simulink model "MdLCtrl_IPC"  (R2019a)
settings: Solver=FixedStepAuto  StartTime=0.0  StopTime=10.0  RelTol=1e-3
values from neighbouring files (symbols this model uses):
  Control = 0.0    [DD_CtrlBaseline.sldd]    (also in DD_MdlCtrl_qLPVMPC.sldd = 0.0
  P_InitAngle = 0.106    [DD_CtrlBaseline.sldd]    (also in ctrl_data.m)
undefined symbols (not defined in the file or in its folder): c1, c2, d1, d2, d3, IPC_An, IPC_K_1P, IPC_KI_1p, IPC_KP_1p, kp_Turm, offest_1p, T_Turmfilter, v_Gen_nenn
settings Model: Creator=ditt_aj  LastModifiedBy=ditt_aj

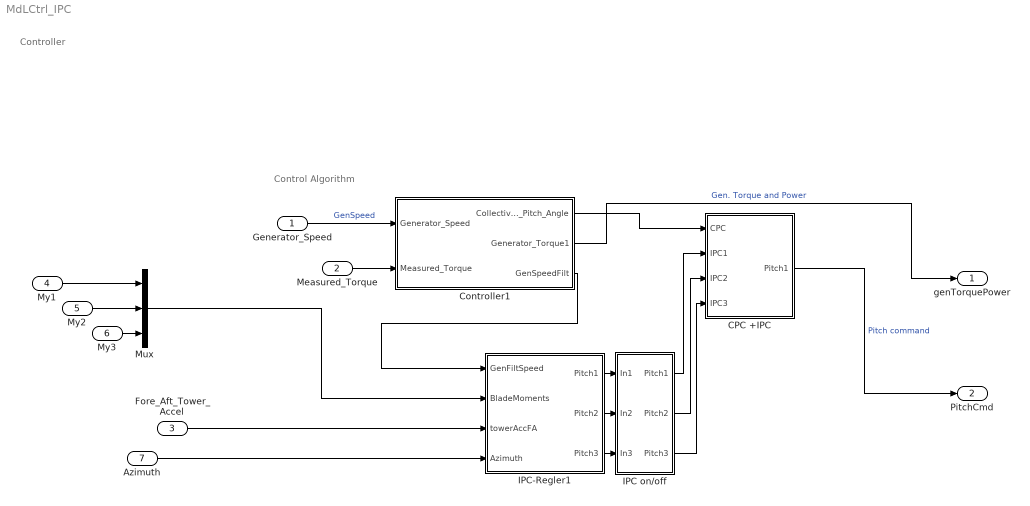
== system MdLCtrl_IPC ==
  note: Control Algorithm
  note: Controller
  Generator_Speed : Inport
  Measured_Torque : Inport  Port=2
  Fore_Aft_Tower_Accel : Inport  Port=3
  My1 : Inport  Port=4
  My2 : Inport  Port=5
  My3 : Inport  Port=6
  Azimuth : Inport  Port=7
  CPC +IPC : Subsystem
  Controller1 : Subsystem
  IPC on/off : Subsystem
  IPC-Regler1 : Subsystem
  Mux : Mux  Inputs=3
  genTorquePower : Outport
  PitchCmd : Outport  Port=2
  wires:
  CPC +IPC/1(Pitch1) -> PitchCmd/1  "Pitch command"
  Controller1/2(Generator_Torque1) -> genTorquePower/1  "Gen. Torque and Power"
  My1/1 -> Mux/1
  My2/1 -> Mux/2
  My3/1 -> Mux/3
  Generator_Speed/1 -> Controller1/1(Generator_Speed)  "GenSpeed"
  Fore_Aft_Tower_Accel/1 -> IPC-Regler1/3(towerAccFA)
  Mux/1 -> IPC-Regler1/2(BladeMoments)
  Azimuth/1 -> IPC-Regler1/4(Azimuth)
  IPC-Regler1/2(Pitch2) -> IPC on/off/2(In2)
  IPC-Regler1/1(Pitch1) -> IPC on/off/1(In1)
  IPC-Regler1/3(Pitch3) -> IPC on/off/3(In3)
  IPC on/off/2(Pitch2) -> CPC +IPC/3(IPC2)
  Controller1/1(Collective_Pitch_Angle) -> CPC +IPC/1(CPC)
  IPC on/off/1(Pitch1) -> CPC +IPC/2(IPC1)
  Controller1/3(GenSpeedFilt) -> IPC-Regler1/1(GenFiltSpeed)
  IPC on/off/3(Pitch3) -> CPC +IPC/4(IPC3)
  Measured_Torque/1 -> Controller1/2(Measured_Torque)

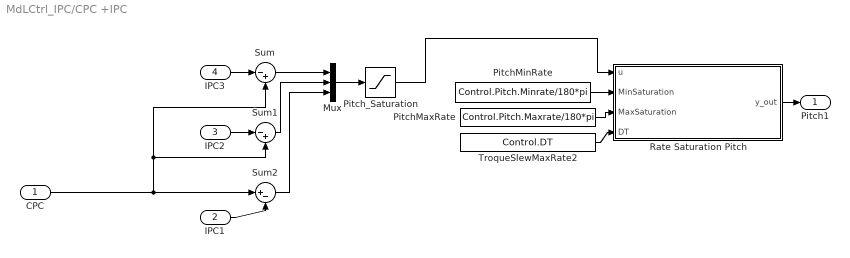
== system MdLCtrl_IPC/CPC +IPC ==
  CPC : Inport
  IPC1 : Inport  Port=2
  IPC2 : Inport  Port=3
  IPC3 : Inport  Port=4
  Mux : Mux  Inputs=3
  PitchMaxRate : Constant  Value=Control.Pitch.Maxrate/180*pi
  PitchMinRate : Constant  Value=Control.Pitch.Minrate/180*pi
  Pitch_Saturation : Saturate  UpperLimit=Control.Pitch.Max*pi/180  LowerLimit=Control.Pitch.Min*pi/180
  Rate Saturation Pitch : MATLAB Function  TreatAsAtomicUnit=on
  Sum : Sum  Inputs=|-+
  Sum1 : Sum  Inputs=|-+
  Sum2 : Sum  Inputs=|+-
  TroqueSlewMaxRate2 : Constant  Value=Control.DT
  Pitch1 : Outport
  wires:
  IPC3/1 -> Sum/1
  IPC2/1 -> Sum1/1
  IPC1/1 -> Sum2/2
  CPC/1 -> Sum1/2, Sum/2, Sum2/1
  TroqueSlewMaxRate2/1 -> Rate Saturation Pitch/4(DT)
  Mux/1 -> Pitch_Saturation/1
  Pitch_Saturation/1 -> Rate Saturation Pitch/1(u)
  PitchMaxRate/1 -> Rate Saturation Pitch/3(MaxSaturation)
  PitchMinRate/1 -> Rate Saturation Pitch/2(MinSaturation)
  Sum/1 -> Mux/1
  Sum1/1 -> Mux/2
  Sum2/1 -> Mux/3
  Rate Saturation Pitch/1(y_out) -> Pitch1/1

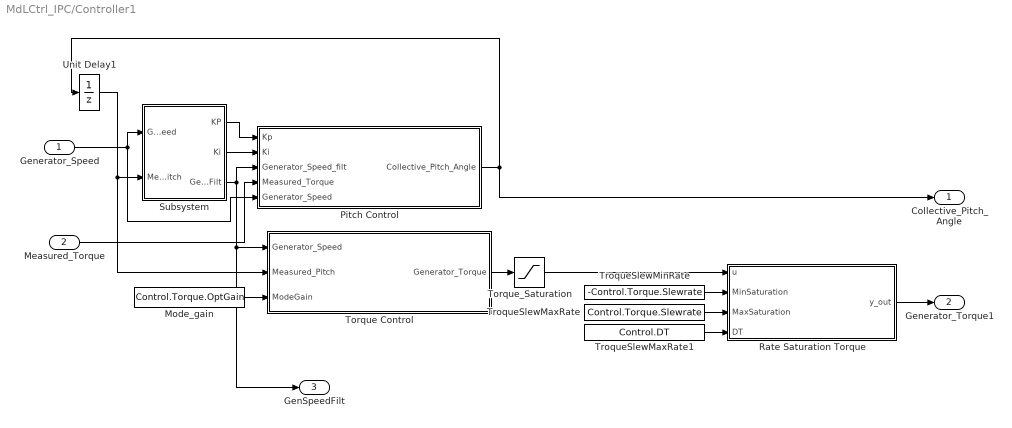
== system MdLCtrl_IPC/Controller1 ==
  Generator_Speed : Inport
  Measured_Torque : Inport  Port=2
  Mode_gain : Constant  Value=Control.Torque.OptGain
  Pitch Control : Subsystem
  Rate Saturation Torque : MATLAB Function  TreatAsAtomicUnit=on
  Subsystem : Subsystem
  Torque Control : Subsystem
  Torque_Saturation : Saturate  UpperLimit=Control.Torque.Limit  LowerLimit=Control.Torque.Min
  TroqueSlewMaxRate : Constant  Value=Control.Torque.Slewrate
  TroqueSlewMaxRate1 : Constant  Value=Control.DT
  TroqueSlewMinRate : Constant  Value=-Control.Torque.Slewrate
  Unit Delay1 : UnitDelay  InitialCondition=P_InitAngle*pi/180  SampleTime=-1  HasFrameUpgradeWarning=on
  Collective_Pitch_Angle : Outport
  Generator_Torque1 : Outport  Port=2
  GenSpeedFilt : Outport  Port=3
  wires:
  Mode_gain/1 -> Torque Control/3(ModeGain)
  Torque_Saturation/1 -> Rate Saturation Torque/1(u)
  TroqueSlewMinRate/1 -> Rate Saturation Torque/2(MinSaturation)
  TroqueSlewMaxRate/1 -> Rate Saturation Torque/3(MaxSaturation)
  TroqueSlewMaxRate1/1 -> Rate Saturation Torque/4(DT)
  Torque Control/1(Generator_Torque) -> Torque_Saturation/1
  Rate Saturation Torque/1(y_out) -> Generator_Torque1/1
  Pitch Control/1(Collective_Pitch_Angle) -> Unit Delay1/1, Collective_Pitch_Angle/1
  Generator_Speed/1 -> Pitch Control/5(Generator_Speed), Subsystem/1(GenSpeed)
  Unit Delay1/1 -> Torque Control/2(Measured_Pitch), Subsystem/2(MesasuredPitch)
  Subsystem/3(GenSpeedFilt) -> GenSpeedFilt/1, Torque Control/1(Generator_Speed), Pitch Control/3(Generator_Speed_filt)
  Subsystem/1(KP) -> Pitch Control/1(Kp)
  Subsystem/2(Ki) -> Pitch Control/2(Ki)
  Measured_Torque/1 -> Pitch Control/4(Measured_Torque)

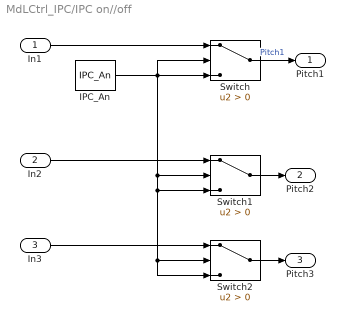
== system MdLCtrl_IPC/IPC on//off ==
  In1 : Inport
  In2 : Inport  Port=2
  In3 : Inport  Port=3
  IPC_An : Constant  Value=IPC_An
  Switch : Switch  Criteria=u2 > Threshold
  Switch1 : Switch  Criteria=u2 > Threshold
  Switch2 : Switch  Criteria=u2 > Threshold
  Pitch1 : Outport
  Pitch2 : Outport  Port=2
  Pitch3 : Outport  Port=3
  wires:
  Switch1/1 -> Pitch2/1
  IPC_An/1 -> Switch1/2, Switch1/3, Switch2/2, Switch2/3, Switch/3, Switch/2
  In3/1 -> Switch2/1
  In1/1 -> Switch/1
  In2/1 -> Switch1/1
  Switch/1 -> Pitch1/1  "Pitch1"
  Switch2/1 -> Pitch3/1

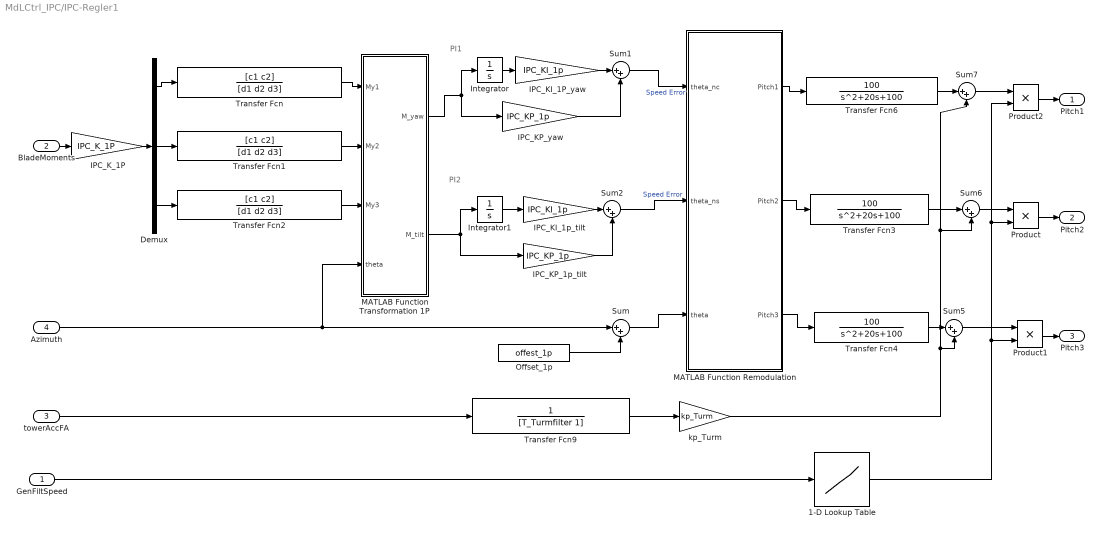
== system MdLCtrl_IPC/IPC-Regler1 ==
  note: PI2
  note: PI1
  GenFiltSpeed : Inport
  BladeMoments : Inport  Port=2
  towerAccFA : Inport  Port=3
  Azimuth : Inport  Port=4
  1-D Lookup Table : Lookup_n-D  NumberOfTableDimensions=1  BreakpointsForDimension1=[0 0.8*v_Gen_nenn 0.9*v_Gen_nenn 1000]  Table=[0 0 1 1]  InternalRulePriority=Speed  RndMeth=Simplest  InputSameDT=on
  Demux : Demux  Outputs=3
  IPC_KI_1P_yaw : Gain  Gain=IPC_KI_1p
  IPC_KI_1p_tilt : Gain  Gain=IPC_KI_1p
  IPC_KP_1p_tilt : Gain  Gain=IPC_KP_1p
  IPC_KP_yaw : Gain  Gain=IPC_KP_1p
  IPC_K_1P : Gain  Gain=IPC_K_1P
  Integrator : Integrator
  Integrator1 : Integrator  LimitOutput=on  UpperSaturationLimit=90  LowerSaturationLimit=-90
  MATLAB Function Remodulation : MATLAB Function  TreatAsAtomicUnit=on
  MATLAB Function Transformation 1P : MATLAB Function  TreatAsAtomicUnit=on
  Offset_1p : Constant  Value=offest_1p
  Product : Product
  Product1 : Product
  Product2 : Product
  Sum{,1..2,5..7} (6 alike) : Sum  Inputs=|++
  Transfer Fcn : TransferFcn  Numerator=[c1 c2]  Denominator=[d1 d2 d3]
  Transfer Fcn1 : TransferFcn  Numerator=[c1 c2]  Denominator=[d1 d2 d3]
  Transfer Fcn2 : TransferFcn  Numerator=[c1 c2]  Denominator=[d1 d2 d3]
  Transfer Fcn3 : TransferFcn  Numerator=100  Denominator=[1 20 100]
  Transfer Fcn4 : TransferFcn  Numerator=100  Denominator=[1 20 100]
  Transfer Fcn6 : TransferFcn  Numerator=100  Denominator=[1 20 100]
  Transfer Fcn9 : TransferFcn  Numerator=1  Denominator=[T_Turmfilter 1]
  kp_Turm : Gain  Gain=kp_Turm
  Pitch1 : Outport
  Pitch2 : Outport  Port=2
  Pitch3 : Outport  Port=3
  wires:
  Azimuth/1 -> MATLAB Function Transformation 1P/4(theta), Sum/1
  kp_Turm/1 -> Sum6/2, Sum7/2, Sum5/2
  Transfer Fcn9/1 -> kp_Turm/1
  Sum5/1 -> Product1/1
  Product2/1 -> Pitch1/1
  1-D Lookup Table/1 -> Product1/2, Product/2, Product2/2
  Product1/1 -> Pitch3/1
  Product/1 -> Pitch2/1
  Sum6/1 -> Product/1
  Sum7/1 -> Product2/1
  GenFiltSpeed/1 -> 1-D Lookup Table/1
  towerAccFA/1 -> Transfer Fcn9/1
  Transfer Fcn6/1 -> Sum7/1
  Transfer Fcn3/1 -> Sum6/1
  Transfer Fcn4/1 -> Sum5/1
  MATLAB Function Remodulation/3(Pitch3) -> Transfer Fcn4/1
  MATLAB Function Remodulation/2(Pitch2) -> Transfer Fcn3/1
  MATLAB Function Remodulation/1(Pitch1) -> Transfer Fcn6/1
  Offset_1p/1 -> Sum/2
  Sum/1 -> MATLAB Function Remodulation/3(theta)
  IPC_K_1P/1 -> Demux/1
  Transfer Fcn2/1 -> MATLAB Function Transformation 1P/3(My3)
  Transfer Fcn/1 -> MATLAB Function Transformation 1P/1(My1)
  Transfer Fcn1/1 -> MATLAB Function Transformation 1P/2(My2)
  BladeMoments/1 -> IPC_K_1P/1
  Demux/3 -> Transfer Fcn2/1
  Demux/2 -> Transfer Fcn1/1
  Demux/1 -> Transfer Fcn/1
  IPC_KI_1P_yaw/1 -> Sum1/1
  IPC_KP_yaw/1 -> Sum1/2
  Integrator/1 -> IPC_KI_1P_yaw/1
  Sum1/1 -> MATLAB Function Remodulation/1(theta_nc)  "Speed Error"
  MATLAB Function Transformation 1P/1(M_yaw) -> Integrator/1, IPC_KP_yaw/1
  Sum2/1 -> MATLAB Function Remodulation/2(theta_ns)  "Speed Error"
  Integrator1/1 -> IPC_KI_1p_tilt/1
  IPC_KP_1p_tilt/1 -> Sum2/2
  IPC_KI_1p_tilt/1 -> Sum2/1
  MATLAB Function Transformation 1P/2(M_tilt) -> Integrator1/1, IPC_KP_1p_tilt/1

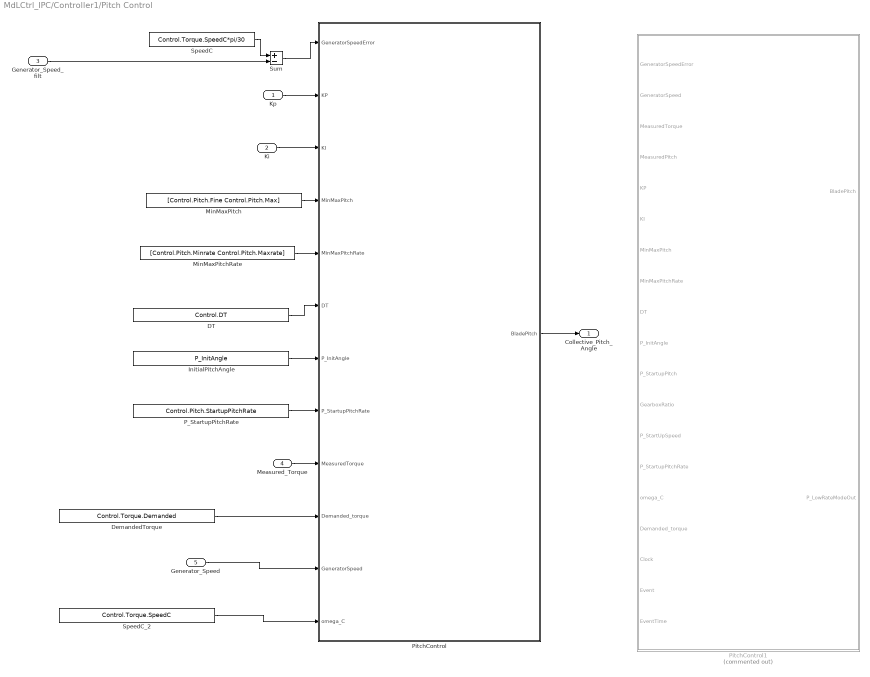
== system MdLCtrl_IPC/Controller1/Pitch Control ==
  Kp : Inport
  Ki : Inport  Port=2
  Generator_Speed_filt : Inport  Port=3
  Measured_Torque : Inport  Port=4
  Generator_Speed : Inport  Port=5
  DT : Constant  Value=Control.DT
  DemandedTorque : Constant  Value=Control.Torque.Demanded
  InitialPitchAngle : Constant  Value=P_InitAngle
  MinMaxPitch : Constant  Value=[Control.Pitch.Fine Control.Pitch.Max]
  MinMaxPitchRate : Constant  Value=[Control.Pitch.Minrate Control.Pitch.Maxrate]
  P_StartupPitchRate : Constant  Value=Control.Pitch.StartupPitchRate
  PitchControl : MATLAB Function  TreatAsAtomicUnit=on
  PitchControl1 : MATLAB Function  Commented=on  TreatAsAtomicUnit=on
  SpeedC : Constant  Value=Control.Torque.SpeedC*pi/30
  SpeedC_2 : Constant  Value=Control.Torque.SpeedC
  Sum : Sum  Inputs=+-
  Collective_Pitch_Angle : Outport
  wires:
  MinMaxPitch/1 -> PitchControl/4(MinMaxPitch)
  MinMaxPitchRate/1 -> PitchControl/5(MinMaxPitchRate)
  PitchControl/1(BladePitch) -> Collective_Pitch_Angle/1
  DT/1 -> PitchControl/6(DT)
  InitialPitchAngle/1 -> PitchControl/7(P_InitAngle)
  P_StartupPitchRate/1 -> PitchControl/8(P_StartupPitchRate)
  SpeedC/1 -> Sum/1
  Sum/1 -> PitchControl/1(GeneratorSpeedError)
  Generator_Speed_filt/1 -> Sum/2
  Kp/1 -> PitchControl/2(KP)
  Ki/1 -> PitchControl/3(KI)
  Measured_Torque/1 -> PitchControl/9(MeasuredTorque)
  SpeedC_2/1 -> PitchControl/12(omega_C)
  Generator_Speed/1 -> PitchControl/11(GeneratorSpeed)
  DemandedTorque/1 -> PitchControl/10(Demanded_torque)

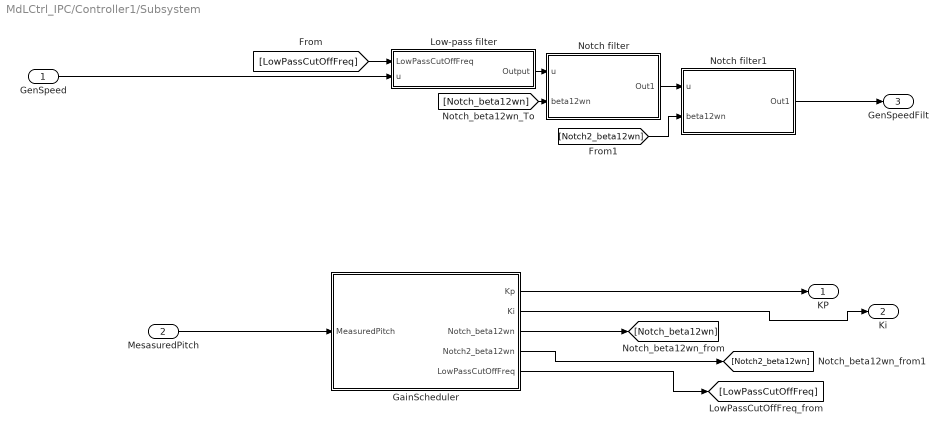
== system MdLCtrl_IPC/Controller1/Subsystem ==
  GenSpeed : Inport
  MesasuredPitch : Inport  Port=2
  GainScheduler : Subsystem
  Low-pass filter : Subsystem
  Notch filter : Subsystem
  Notch filter1 : Subsystem
  KP : Outport
  Ki : Outport  Port=2
  GenSpeedFilt : Outport  Port=3
  wires:
  [LowPassCutOffFreq] -> Low-pass filter/1(LowPassCutOffFreq)
  Notch filter/1(Out1) -> Notch filter1/1(u)
  Low-pass filter/1(Output) -> Notch filter/1(u)
  GainScheduler/3(Notch_beta12wn) -> [Notch_beta12wn]
  GainScheduler/5(LowPassCutOffFreq) -> [LowPassCutOffFreq]
  GainScheduler/2(Ki) -> Ki/1
  [Notch_beta12wn] -> Notch filter/2(beta12wn)
  GainScheduler/4(Notch2_beta12wn) -> [Notch2_beta12wn]
  [Notch2_beta12wn] -> Notch filter1/2(beta12wn)
  MesasuredPitch/1 -> GainScheduler/1(MeasuredPitch)
  GainScheduler/1(Kp) -> KP/1
  Notch filter1/1(Out1) -> GenSpeedFilt/1
  GenSpeed/1 -> Low-pass filter/2(u)

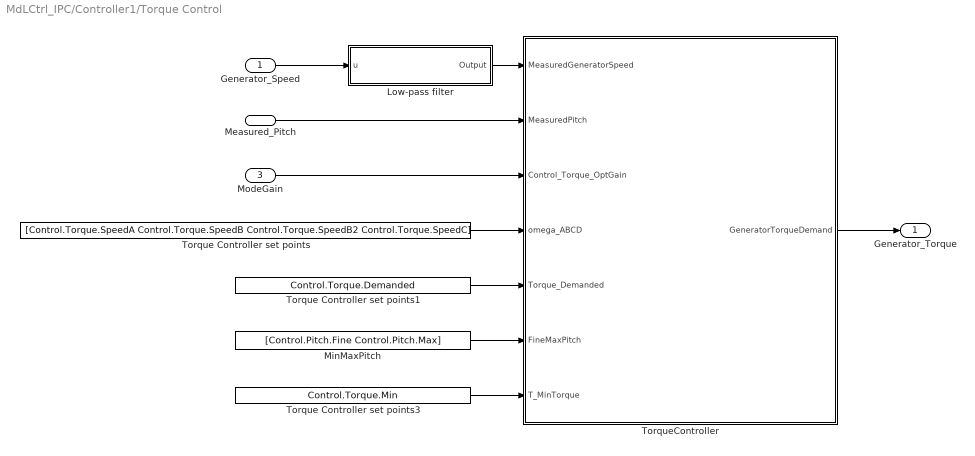
== system MdLCtrl_IPC/Controller1/Torque Control ==
  Generator_Speed : Inport
  Measured_Pitch : Inport  Port=2
  ModeGain : Inport  Port=3
  Low-pass filter : Subsystem
  MinMaxPitch : Constant  Value=[Control.Pitch.Fine Control.Pitch.Max]
  Torque Controller set points : Constant  Value=[Control.Torque.SpeedA Control.Torque.SpeedB Control.Torque.SpeedB2 Control.Torque.SpeedC]
  Torque Controller set points1 : Constant  Value=Control.Torque.Demanded
  Torque Controller set points3 : Constant  Value=Control.Torque.Min
  TorqueController : MATLAB Function  TreatAsAtomicUnit=on
  Generator_Torque : Outport
  wires:
  Generator_Speed/1 -> Low-pass filter/1(u)
  TorqueController/1(GeneratorTorqueDemand) -> Generator_Torque/1
  Measured_Pitch/1 -> TorqueController/2(MeasuredPitch)
  ModeGain/1 -> TorqueController/3(Control_Torque_OptGain)
  Torque Controller set points/1 -> TorqueController/4(omega_ABCD)
  Low-pass filter/1(Output) -> TorqueController/1(MeasuredGeneratorSpeed)
  Torque Controller set points3/1 -> TorqueController/7(T_MinTorque)
  MinMaxPitch/1 -> TorqueController/6(FineMaxPitch)
  Torque Controller set points1/1 -> TorqueController/5(Torque_Demanded)

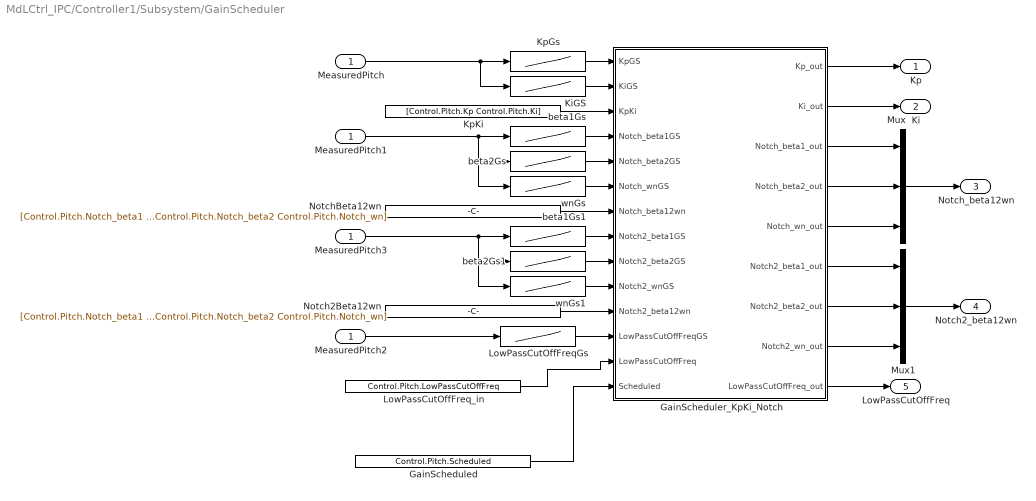
== system MdLCtrl_IPC/Controller1/Subsystem/GainScheduler ==
  MeasuredPitch : Inport
  GainScheduled : Constant  Value=Control.Pitch.Scheduled
  GainScheduler_KpKi_Notch : MATLAB Function  TreatAsAtomicUnit=on
  KiGS : Lookup_n-D  NumberOfTableDimensions=1  BreakpointsForDimension1=Control.Pitch.ScheduledPitchAngles  Table=Control.Pitch.KiGS  ExtrapMethod=Clip  UseLastTableValue=on  InternalRulePriority=Speed  RndMeth=Simplest  InputSameDT=on
  KpGs : Lookup_n-D  NumberOfTableDimensions=1  BreakpointsForDimension1=Control.Pitch.ScheduledPitchAngles  Table=Control.Pitch.KpGS  ExtrapMethod=Clip  UseLastTableValue=on  InternalRulePriority=Speed  RndMeth=Simplest  InputSameDT=on
  KpKi : Constant  Value=[Control.Pitch.Kp Control.Pitch.Ki]
  LowPassCutOffFreqGs : Lookup_n-D  NumberOfTableDimensions=1  BreakpointsForDimension1=Control.Pitch.ScheduledPitchAngles  Table=Control.Pitch.LowPassCutOffFreqGS  ExtrapMethod=Clip  UseLastTableValue=on  InternalRulePriority=Speed  RndMeth=Simplest  InputSameDT=on
  LowPassCutOffFreq_in : Constant  Value=Control.Pitch.LowPassCutOffFreq
  MeasuredPitch1 : InportShadow
  MeasuredPitch2 : InportShadow
  MeasuredPitch3 : InportShadow
  Mux : Mux  Inputs=3
  Mux1 : Mux  Inputs=3
  Notch2Beta12wn : Constant  Value=[Control.Pitch.Notch_beta1 Control.Pitch.Notch_beta2 Control.Pitch.Notch_wn]
  NotchBeta12wn : Constant  Value=[Control.Pitch.Notch_beta1 Control.Pitch.Notch_beta2 Control.Pitch.Notch_wn]
  beta1Gs : Lookup_n-D  NumberOfTableDimensions=1  BreakpointsForDimension1=Control.Pitch.ScheduledPitchAngles  Table=Control.Pitch.Notch_beta1GS  ExtrapMethod=Clip  UseLastTableValue=on  InternalRulePriority=Speed  RndMeth=Simplest  InputSameDT=on
  beta1Gs1 : Lookup_n-D  NumberOfTableDimensions=1  BreakpointsForDimension1=Control.Pitch.ScheduledPitchAngles  Table=Control.Pitch.Notch2_beta1GS  ExtrapMethod=Clip  UseLastTableValue=on  InternalRulePriority=Speed  RndMeth=Simplest  InputSameDT=on
  beta2Gs : Lookup_n-D  NumberOfTableDimensions=1  BreakpointsForDimension1=Control.Pitch.ScheduledPitchAngles  Table=Control.Pitch.Notch_beta2GS  ExtrapMethod=Clip  UseLastTableValue=on  InternalRulePriority=Speed  RndMeth=Simplest  InputSameDT=on
  beta2Gs1 : Lookup_n-D  NumberOfTableDimensions=1  BreakpointsForDimension1=Control.Pitch.ScheduledPitchAngles  Table=Control.Pitch.Notch2_beta2GS  ExtrapMethod=Clip  UseLastTableValue=on  InternalRulePriority=Speed  RndMeth=Simplest  InputSameDT=on
  wnGs : Lookup_n-D  NumberOfTableDimensions=1  BreakpointsForDimension1=Control.Pitch.ScheduledPitchAngles  Table=Control.Pitch.Notch_wnGS  ExtrapMethod=Clip  UseLastTableValue=on  InternalRulePriority=Speed  RndMeth=Simplest  InputSameDT=on
  wnGs1 : Lookup_n-D  NumberOfTableDimensions=1  BreakpointsForDimension1=Control.Pitch.ScheduledPitchAngles  Table=Control.Pitch.Notch2_wnGS  ExtrapMethod=Clip  UseLastTableValue=on  InternalRulePriority=Speed  RndMeth=Simplest  InputSameDT=on
  Kp : Outport
  Ki : Outport  Port=2
  Notch_beta12wn : Outport  Port=3
  Notch2_beta12wn : Outport  Port=4
  LowPassCutOffFreq : Outport  Port=5
  wires:
  MeasuredPitch/1 -> KiGS/1, KpGs/1
  GainScheduled/1 -> GainScheduler_KpKi_Notch/14(Scheduled)
  GainScheduler_KpKi_Notch/2(Ki_out) -> Ki/1
  KpKi/1 -> GainScheduler_KpKi_Notch/3(KpKi)
  KpGs/1 -> GainScheduler_KpKi_Notch/1(KpGS)
  KiGS/1 -> GainScheduler_KpKi_Notch/2(KiGS)
  GainScheduler_KpKi_Notch/1(Kp_out) -> Kp/1
  GainScheduler_KpKi_Notch/3(Notch_beta1_out) -> Mux/1
  GainScheduler_KpKi_Notch/4(Notch_beta2_out) -> Mux/2
  GainScheduler_KpKi_Notch/5(Notch_wn_out) -> Mux/3
  NotchBeta12wn/1 -> GainScheduler_KpKi_Notch/7(Notch_beta12wn)
  MeasuredPitch1/1 -> wnGs/1, beta2Gs/1, beta1Gs/1
  beta1Gs/1 -> GainScheduler_KpKi_Notch/4(Notch_beta1GS)
  beta2Gs/1 -> GainScheduler_KpKi_Notch/5(Notch_beta2GS)
  wnGs/1 -> GainScheduler_KpKi_Notch/6(Notch_wnGS)
  Mux/1 -> Notch_beta12wn/1
  MeasuredPitch2/1 -> LowPassCutOffFreqGs/1
  LowPassCutOffFreqGs/1 -> GainScheduler_KpKi_Notch/12(LowPassCutOffFreqGS)
  LowPassCutOffFreq_in/1 -> GainScheduler_KpKi_Notch/13(LowPassCutOffFreq)
  GainScheduler_KpKi_Notch/9(LowPassCutOffFreq_out) -> LowPassCutOffFreq/1
  GainScheduler_KpKi_Notch/7(Notch2_beta2_out) -> Mux1/2
  Mux1/1 -> Notch2_beta12wn/1
  GainScheduler_KpKi_Notch/6(Notch2_beta1_out) -> Mux1/1
  GainScheduler_KpKi_Notch/8(Notch2_wn_out) -> Mux1/3
  MeasuredPitch3/1 -> wnGs1/1, beta2Gs1/1, beta1Gs1/1
  beta1Gs1/1 -> GainScheduler_KpKi_Notch/8(Notch2_beta1GS)
  beta2Gs1/1 -> GainScheduler_KpKi_Notch/9(Notch2_beta2GS)
  wnGs1/1 -> GainScheduler_KpKi_Notch/10(Notch2_wnGS)
  Notch2Beta12wn/1 -> GainScheduler_KpKi_Notch/11(Notch2_beta12wn)

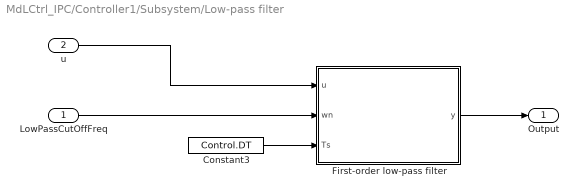
== system MdLCtrl_IPC/Controller1/Subsystem/Low-pass filter ==
  LowPassCutOffFreq : Inport
  u : Inport  Port=2
  Constant3 : Constant  Value=Control.DT
  First-order low-pass filter : MATLAB Function  TreatAsAtomicUnit=on
  Output : Outport
  wires:
  First-order low-pass filter/1(y) -> Output/1
  Constant3/1 -> First-order low-pass filter/3(Ts)
  LowPassCutOffFreq/1 -> First-order low-pass filter/2(wn)
  u/1 -> First-order low-pass filter/1(u)

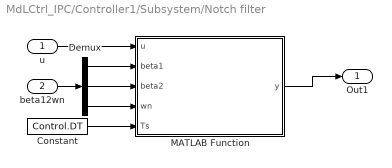
== system MdLCtrl_IPC/Controller1/Subsystem/Notch filter ==
  u : Inport
  beta12wn : Inport  Port=2
  Constant : Constant  Value=Control.DT
  Demux : Demux  Outputs=3
  MATLAB Function : MATLAB Function  TreatAsAtomicUnit=on
  Out1 : Outport
  wires:
  MATLAB Function/1(y) -> Out1/1
  Demux/1 -> MATLAB Function/2(beta1)
  Demux/2 -> MATLAB Function/3(beta2)
  Demux/3 -> MATLAB Function/4(wn)
  beta12wn/1 -> Demux/1
  u/1 -> MATLAB Function/1(u)
  Constant/1 -> MATLAB Function/5(Ts)

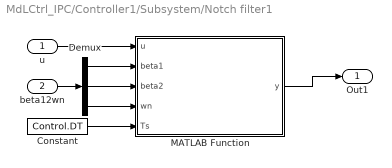
== system MdLCtrl_IPC/Controller1/Subsystem/Notch filter1 ==
  u : Inport
  beta12wn : Inport  Port=2
  Constant : Constant  Value=Control.DT
  Demux : Demux  Outputs=3
  MATLAB Function : MATLAB Function  TreatAsAtomicUnit=on
  Out1 : Outport
  wires:
  MATLAB Function/1(y) -> Out1/1
  Demux/1 -> MATLAB Function/2(beta1)
  Demux/2 -> MATLAB Function/3(beta2)
  Demux/3 -> MATLAB Function/4(wn)
  beta12wn/1 -> Demux/1
  u/1 -> MATLAB Function/1(u)
  Constant/1 -> MATLAB Function/5(Ts)

== system MdLCtrl_IPC/Controller1/Torque Control/Low-pass filter ==
  u : Inport
  Constant1 : Constant  Value=Control.Torque.LowPassCutOffFreq
  Constant3 : Constant  Value=Control.DT
  First-order low-pass filter : MATLAB Function  TreatAsAtomicUnit=on
  Output : Outport
  wires:
  Constant3/1 -> First-order low-pass filter/3(Ts)
  u/1 -> First-order low-pass filter/1(u)
  First-order low-pass filter/1(y) -> Output/1
  Constant1/1 -> First-order low-pass filter/2(wn)

== matlab function MdLCtrl_IPC/Controller1/Pitch Control/PitchControl1 ==
  settings: updateMethod=DISCRETE  sampleTime=Control.DT
  data: GeneratorSpeedError input; GeneratorSpeed input; MeasuredTorque input; MeasuredPitch input; BladePitch output; KP input; KI input; MinMaxPitch input; MinMaxPitchRate input; DT input; P_InitAngle input; P_StartupPitch input; GearboxRatio input; P_StartUpSpeed input; P_StartupPitchRate input; omega_C input; Demanded_torque input; Clock input; P_LowRateModeOut output boolean; Event input; EventTime input
function [BladePitch, P_LowRateModeOut]  = PitchControl(GeneratorSpeedError, GeneratorSpeed, MeasuredTorque, MeasuredPitch, KP, KI, MinMaxPitch, MinMaxPitchRate, DT, P_InitAngle, P_StartupPitch, GearboxRatio, P_StartUpSpeed, P_StartupPitchRate, omega_C, Demanded_torque, Clock, Event, EventTime)
persistent I_term PI_term_old P_LowRateMode P_LowRateMode_old

%Initialize all persistent variables
if isempty(I_term)
    I_term = (P_InitAngle*pi/180);
    PI_term_old = (P_InitAngle*pi/180);
    P_LowRateMode = true;
    P_LowRateMode_old = true; %Used to detect change from start-up/below-rated to above-rated operation mode
end

%Event handling part
if (Event == 2 && Clock >= EventTime) || (Event == 5 && Clock >= EventTime) %Grid loss, emergency shutdown
    P_LowRateMode = false;
    P_MinPitchSat = MinMaxPitch(2)*pi/180;
elseif (Event == 4 && Clock >= EventTime) % Normal shutdown
    P_LowRateMode = true;
    P_MinPitchSat = MinMaxPitch(2)*pi/180;
elseif Event == 7 || Event == 6 % Idling and parked mode
    P_MinPitchSat = MinMaxPitch(2)*pi/180;
elseif MeasuredTorque > Demanded_torque*0.99 || GeneratorSpeed > omega_C*(pi/30) % Above-rated operating mode
    P_LowRateMode = false;
    P_MinPitchSat = MinMaxPitch(1)*pi/180;
    if P_LowRateMode ~= P_LowRateMode_old % On switching event between below-rated to above rated, reinitialize the integral term to ensure smooth transition
        I_term = MeasuredPitch;
    end
elseif Event == 3 || GeneratorSpeed < P_StartUpSpeed*GearboxRatio*(pi/30) % Normal startup 
    if Event == 3 && Clock < EventTime
        P_LowRateMode = true;
        P_MinPitchSat = MinMaxPitch(2)*pi/180;
    elseif (Event == 3 && Clock >= EventTime) && (GeneratorSpeed < P_StartUpSpeed*GearboxRatio*(pi/30))
        P_LowRateMode = true;
        P_MinPitchSat = P_StartupPitch*pi/180;
    else
        P_LowRateMode = true;
        P_MinPitchSat = MinMaxPitch(1)*pi/180;
    end
else
    P_MinPitchSat = MinMaxPitch(1)*pi/180;
end
 
% Pitch controller, KP and KI are constant or gain-scheduled, depending on
% input. Integral term is saturated, lower bound is variable and depends on
% event or operatinig mode.
P_term = KP*GeneratorSpeedError;
I_term = I_term + KI*GeneratorSpeedError*DT;
I_term = min(max(I_term,P_MinPitchSat), MinMaxPitch(2)*pi/180);

PI_term = P_term + I_term;
PI_term_sat = min(max(PI_term,P_MinPitchSat), MinMaxPitch(2)*pi/180);

% Calculate and limit pitch rate. Limit on rate is subject to event or
% operating mode.
PitchRate = (PI_term_sat - PI_term_old)/DT;
if P_LowRateMode
    PitchRate = min(max(PitchRate, -P_StartupPitchRate*pi/180), P_StartupPitchRate*pi/180);
else
    PitchRate = min(max(PitchRate, MinMaxPitchRate(1)*pi/180), MinMaxPitchRate(2)*pi/180);
end
BladePitch = PI_term_old + PitchRate*DT;

% Write variables to persistent variables and/or outputs
PI_term_old = BladePitch;
P_LowRateModeOut = P_LowRateMode;
P_LowRateMode_old = P_LowRateMode;
end

== matlab function MdLCtrl_IPC/CPC +IPC/Rate Saturation Pitch ==
  settings: updateMethod=DISCRETE
  data: u input; MinSaturation input; y_out output; MaxSaturation input; DT input
function y_out = fcn(u, MinSaturation, MaxSaturation, DT)
persistent y

if isempty(y)
    y = u;
end

rate = (u-y)/DT;
rate = min(max(rate, MinSaturation), MaxSaturation);

y = y + rate*DT;
y_out = y;

== matlab function MdLCtrl_IPC/IPC-Regler1/MATLAB Function Remodulation ==
  data: theta_nc input; Pitch1 output; theta_ns input; Pitch2 output; Pitch3 output; theta input
function [Pitch1,Pitch2,Pitch3] = remodulation(theta_nc,theta_ns,theta)
%#codegen
Pitch=[cos(theta)          sin(theta);...
       cos(theta+2*pi/3) sin(theta+2*pi/3);...
       cos(theta+4*pi/3) sin(theta+4*pi/3)] *[theta_nc;theta_ns];
   
   Pitch1 = Pitch(1);
   Pitch2 = Pitch(2);
   Pitch3 = Pitch(3);

== matlab function MdLCtrl_IPC/IPC-Regler1/MATLAB Function Transformation 1P ==
  data: My1 input; M_yaw output; My2 input; My3 input; M_tilt output; theta input
function [M_yaw,M_tilt] = demodulation(My1,My2,My3,theta)
% Coleman Transformation: D-q transformation of blade moments
% https://en.wikipedia.org/wiki/Direct%E2%80%93quadrature%E2%80%93zero_transformation
% 
% Inputs
%  - Blade root moments in rotating frame: My1,My2,My3
%  - Azimuth
% Outputs 
%  - M_Yaw: Mnc, moment around tower, Axis positiv upwards
%  - M_tilt: Mns, quadrature-axis (um y (Achse weder in Windrichtung  noch nach oben))

%#codegen
Mout=[cos(theta) cos((theta+2*pi/3)) cos((theta+4*pi/3));...
      sin(theta) sin((theta+2*pi/3)) sin((theta+4*pi/3))] *[My1;My2;My3];

M_yaw  = 2/3*Mout(1);
M_tilt = 2/3*Mout(2);

== matlab function MdLCtrl_IPC/Controller1/Subsystem/GainScheduler/GainScheduler_KpKi_Notch ==
  data: KpGS input; KiGS input; Kp_out output; KpKi input; Notch_beta1GS input; Notch_beta2GS input; Notch_wnGS input; Notch_beta12wn input; Notch2_beta1GS input; Notch2_beta2GS input; Notch2_wnGS input; Notch2_beta12wn input; LowPassCutOffFreqGS input; LowPassCutOffFreq input; Scheduled input; Ki_out output; Notch_beta1_out output; Notch_beta2_out output; Notch_wn_out output; Notch2_beta1_out output; Notch2_beta2_out output; Notch2_wn_out output; LowPassCutOffFreq_out output
function [Kp_out, Ki_out, Notch_beta1_out, Notch_beta2_out, Notch_wn_out, Notch2_beta1_out, Notch2_beta2_out, Notch2_wn_out, LowPassCutOffFreq_out] = fcn(KpGS, KiGS, KpKi, Notch_beta1GS, Notch_beta2GS, Notch_wnGS, Notch_beta12wn, Notch2_beta1GS, Notch2_beta2GS, Notch2_wnGS, Notch2_beta12wn, LowPassCutOffFreqGS, LowPassCutOffFreq, Scheduled)

if Scheduled > 0.5
    Kp_out = KpGS;
    Ki_out = KiGS;
    Notch_beta1_out = Notch_beta1GS;
    Notch_beta2_out = Notch_beta2GS;
    Notch_wn_out = Notch_wnGS;
    Notch2_beta1_out = Notch2_beta1GS;
    Notch2_beta2_out = Notch2_beta2GS;
    Notch2_wn_out = Notch2_wnGS;
    LowPassCutOffFreq_out = LowPassCutOffFreqGS;
else
    Kp_out = KpKi(1);
    Ki_out = KpKi(2);
    Notch_beta1_out = Notch_beta12wn(1);
    Notch_beta2_out = Notch_beta12wn(2);
    Notch_wn_out = Notch_beta12wn(3);
    Notch2_beta1_out = Notch2_beta12wn(1);
    Notch2_beta2_out = Notch2_beta12wn(2);
    Notch2_wn_out = Notch2_beta12wn(3);
    LowPassCutOffFreq_out = LowPassCutOffFreq;
end

== matlab function MdLCtrl_IPC/Controller1/Subsystem/Low-pass filter/First-order low-pass filter ==
  settings: updateMethod=DISCRETE
  data: u input; wn input; y output; Ts input
function y = FirstLPF(u, wn, Ts)

persistent y_prev1 u_prev1

if isempty(u_prev1)
    y_prev1 = u;
    u_prev1 = u;
end

y = (Ts*wn*u + Ts*wn*u_prev1 - (Ts*wn-2.0)*y_prev1)/(Ts*wn+2.0);

u_prev1   = u;
y_prev1  = y;

== matlab function MdLCtrl_IPC/Controller1/Subsystem/Notch filter/MATLAB Function ==
  data: u input; beta1 input; beta2 input; wn input; y output; Ts input
function y = NotchFilter(u, beta1, beta2, wn, Ts)

persistent u_prev1 u_prev2 y_prev1 y_prev2
if isempty(u_prev1)
    u_prev1 = u;
    u_prev2 = u;
    y_prev1 = u;
    y_prev2 = u;
end

if any([beta1 beta2 wn] == 0)
    y = u;
else
    % Prepare filter elements from current input
    K = 2/Ts;
    Part1 = (K^2 + 2*wn*beta1 * K + wn^2) / (K^2 + 2*wn*beta2 * K + wn^2);
    Part2 = (2 * wn^2 - 2 * K^2)  / (K^2 + 2*wn*beta2 * K + wn^2);
    Part3 = (K^2 - 2*wn*beta1 * K + wn^2) / (K^2 + 2*wn*beta2 * K + wn^2);
    Part4 = (2 * wn^2 - 2 * K^2)  / (K^2 + 2*wn*beta2 * K + wn^2);
    Part5 = (K^2 - 2*wn*beta2* K + wn^2)/ (K^2 + 2*wn*beta2 * K + wn^2);
    
    % Compute filter output
    y = Part1*u + Part2*u_prev1 + Part3*u_prev2 - Part4*y_prev1 - Part5*y_prev2;
    
    % Save signals for next time step
    u_prev2 = u_prev1;
    u_prev1 = u;
    
    y_prev2 = y_prev1;
    y_prev1 = y;
end

== matlab function MdLCtrl_IPC/Controller1/Subsystem/Notch filter1/MATLAB Function ==
  data: u input; beta1 input; beta2 input; wn input; y output; Ts input
function y = NotchFilter(u, beta1, beta2, wn, Ts)

persistent u_prev1 u_prev2 y_prev1 y_prev2
if isempty(u_prev1)
    u_prev1 = u;
    u_prev2 = u;
    y_prev1 = u;
    y_prev2 = u;
end

if any([beta1 beta2 wn] == 0)
    y = u;
else
    % Prepare filter elements from current input
    K = 2/Ts;
    Part1 = (K^2 + 2*wn*beta1 * K + wn^2) / (K^2 + 2*wn*beta2 * K + wn^2);
    Part2 = (2 * wn^2 - 2 * K^2)  / (K^2 + 2*wn*beta2 * K + wn^2);
    Part3 = (K^2 - 2*wn*beta1 * K + wn^2) / (K^2 + 2*wn*beta2 * K + wn^2);
    Part4 = (2 * wn^2 - 2 * K^2)  / (K^2 + 2*wn*beta2 * K + wn^2);
    Part5 = (K^2 - 2*wn*beta2* K + wn^2)/ (K^2 + 2*wn*beta2 * K + wn^2);
    
    % Compute filter output
    y = Part1*u + Part2*u_prev1 + Part3*u_prev2 - Part4*y_prev1 - Part5*y_prev2;
    
    % Save signals for next time step
    u_prev2 = u_prev1;
    u_prev1 = u;
    
    y_prev2 = y_prev1;
    y_prev1 = y;
end

== matlab function MdLCtrl_IPC/Controller1/Pitch Control/PitchControl ==
  settings: updateMethod=DISCRETE  sampleTime=Control.DT
  data: GeneratorSpeedError input; BladePitch output; KP input; KI input; MinMaxPitch input; MinMaxPitchRate input; DT input; P_InitAngle input; P_StartupPitchRate input; MeasuredTorque input; Demanded_torque input; GeneratorSpeed input; omega_C input
function BladePitch = PitchControl(GeneratorSpeedError, KP, KI, MinMaxPitch, MinMaxPitchRate, DT, P_InitAngle,P_StartupPitchRate, MeasuredTorque,Demanded_torque,GeneratorSpeed,omega_C)
persistent I_term PI_term_old P_LowRateMode P_LowRateMode_old

%Initialize all persistent variables
if isempty(I_term)
    I_term = (P_InitAngle*pi/180);
    PI_term_old = (P_InitAngle*pi/180);
    P_LowRateMode = true;
    P_LowRateMode_old = true; %Used to detect change from start-up/below-rated to above-rated operation mode
end

%Event handling part
% if (Event == 2 && Clock >= EventTime) || (Event == 5 && Clock >= EventTime) %Grid loss, emergency shutdown
%     P_LowRateMode = false;
%     P_MinPitchSat = MinMaxPitch(2)*pi/180;
% elseif (Event == 4 && Clock >= EventTime) % Normal shutdown
%     P_LowRateMode = true;
%     P_MinPitchSat = MinMaxPitch(2)*pi/180;
% elseif Event == 7 || Event == 6 % Idling and parked mode
%     P_MinPitchSat = MinMaxPitch(2)*pi/180;
if MeasuredTorque > Demanded_torque*0.99 || GeneratorSpeed > omega_C*(pi/30) % Above-rated operating mode
    P_LowRateMode = false;
    P_MinPitchSat = MinMaxPitch(1)*pi/180;
    if P_LowRateMode ~= P_LowRateMode_old % On switching event between below-rated to above rated, reinitialize the integral term to ensure smooth transition
        I_term = MeasuredPitch;
    end
% elseif Event == 3 || GeneratorSpeed < P_StartUpSpeed*GearboxRatio*(pi/30) % Normal startup 
%     if Event == 3 && Clock < EventTime
%         P_LowRateMode = true;
%         P_MinPitchSat = MinMaxPitch(2)*pi/180;
%     elseif (Event == 3 && Clock >= EventTime) && (GeneratorSpeed < P_StartUpSpeed*GearboxRatio*(pi/30))
%         P_LowRateMode = true;
%         P_MinPitchSat = P_StartupPitch*pi/180;
%     else
%         P_LowRateMode = true;
%         P_MinPitchSat = MinMaxPitch(1)*pi/180;
%     end
else
    P_MinPitchSat = MinMaxPitch(1)*pi/180;
end
 
% Pitch controller, KP and KI are constant or gain-scheduled, depending on
% input. Integral term is saturated, lower bound is variable and depends on
% event or operatinig mode.
P_term = KP*GeneratorSpeedError;
I_term = I_term + KI*GeneratorSpeedError*DT;
I_term = min(max(I_term,P_MinPitchSat), MinMaxPitch(2)*pi/180);

PI_term = P_term + I_term;
PI_term_sat = min(max(PI_term,P_MinPitchSat), MinMaxPitch(2)*pi/180);

% Calculate and limit pitch rate. Limit on rate is subject to event or
% operating mode.
PitchRate = (PI_term_sat - PI_term_old)/DT;
if P_LowRateMode
    PitchRate = min(max(PitchRate, -P_StartupPitchRate*pi/180), P_StartupPitchRate*pi/180);
else
    PitchRate = min(max(PitchRate, MinMaxPitchRate(1)*pi/180), MinMaxPitchRate(2)*pi/180);
end
BladePitch = PI_term_old + PitchRate*DT;

% Write variables to persistent variables and/or outputs
PI_term_old = BladePitch;
% P_LowRateModeOut = P_LowRateMode;
P_LowRateMode_old = P_LowRateMode;
end

== matlab function MdLCtrl_IPC/Controller1/Rate Saturation Torque ==
  settings: updateMethod=DISCRETE
  data: u input; MinSaturation input; y_out output; MaxSaturation input; DT input
function y_out = fcn(u, MinSaturation, MaxSaturation, DT)
persistent y

if isempty(y)
    y = u;
end

rate = (u-y)/DT;
rate = min(max(rate, MinSaturation), MaxSaturation);

y = y + rate*DT;
y_out = y;

== matlab function MdLCtrl_IPC/Controller1/Torque Control/Low-pass filter/First-order low-pass filter ==
  settings: updateMethod=DISCRETE
  data: u input; wn input; y output; Ts input
function y = FirstLPF(u, wn, Ts)

persistent y_prev1 u_prev1

if isempty(u_prev1)
    y_prev1 = u;
    u_prev1 = u;
end

y = (Ts*wn*u + Ts*wn*u_prev1 - (Ts*wn-2.0)*y_prev1)/(Ts*wn+2.0);

u_prev1   = u;
y_prev1  = y;

== matlab function MdLCtrl_IPC/Controller1/Torque Control/TorqueController ==
  data: GeneratorTorqueDemand output; MeasuredGeneratorSpeed input; MeasuredPitch input; Control_Torque_OptGain input; omega_ABCD input size=[1 4]; Torque_Demanded input; FineMaxPitch input; T_MinTorque input
function GeneratorTorqueDemand  = TorqueController(MeasuredGeneratorSpeed, MeasuredPitch, Control_Torque_OptGain, omega_ABCD, Torque_Demanded, FineMaxPitch, T_MinTorque)

% Calculate generator torque setpoint according to the feedforward wind
% turbine control law T = K*\omega^2
GeneratorTorqueDemand = max(min(Control_Torque_OptGain*MeasuredGeneratorSpeed^2, Torque_Demanded), T_MinTorque);

% Calculate torques at beginning and end of CP_max operation
TorqueOmegaB = Control_Torque_OptGain*(omega_ABCD(2)*pi/30)^2;
TorqueOmegaC = Control_Torque_OptGain*(omega_ABCD(3)*pi/30)^2;

% Apply maximum demanded torque when pitch is 1 degree above fine-pitch and
% the wind turbine is not in start-up mode.
% if (Event == 5 && Clock >= EventTime) && (MeasuredPitch > (FineMaxPitch(2) - 1.0)*pi/180) %Emergency shutdown
%     GeneratorTorqueDemand = 0.0;
% else
    
if MeasuredPitch > (FineMaxPitch(1) + 1.0)*pi/180 % && P_StartupMode == false
    GeneratorTorqueDemand = Torque_Demanded;
elseif MeasuredGeneratorSpeed < omega_ABCD(1)*pi/30
    GeneratorTorqueDemand = T_MinTorque;
elseif MeasuredGeneratorSpeed < omega_ABCD(2)*pi/30
    GeneratorTorqueDemand = (TorqueOmegaB - T_MinTorque)/((omega_ABCD(2) - omega_ABCD(1))*pi/30)*(MeasuredGeneratorSpeed - omega_ABCD(1)*pi/30) + T_MinTorque;
elseif MeasuredGeneratorSpeed >= omega_ABCD(3)*pi/30
    GeneratorTorqueDemand = (Torque_Demanded - TorqueOmegaC)/((omega_ABCD(4) - omega_ABCD(3))*pi/30)*(MeasuredGeneratorSpeed - omega_ABCD(3)*pi/30) + TorqueOmegaC;
end
